simulink model "casper_counter"  (R2019a)
settings: Solver=VariableStepAuto  StartTime=0.0  StopTime=10.0  RelTol=1e-3
libraries: xbsIndex_r4 x2, xps_library x1
settings Model: Creator=talon  LastModifiedBy=talon

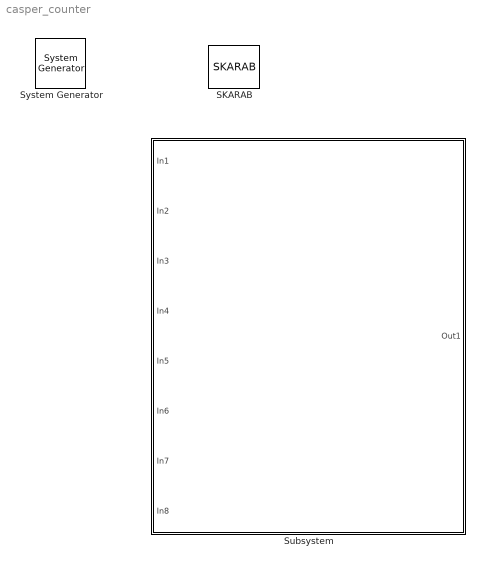
== system casper_counter ==
  " System Generator" : xbsIndex_r4/ System Generator  Tag=genX  xilinxfamily=kintex7  part=xc7k325t  speed=-3  package=fbg676  synthesis_tool=Vivado  clock_wrapper=Clock Enables  directory=./netlist  proj_type=Vivado  Synth_file=Vivado Synthesis Defaults  Impl_file=Vivado Implementation Defaults  testbench=off  simulink_period=1  sysclk_period=10  dcm_input_clock_period=10  incr_netlist=off  trim_vbits=Everywhere in SubSystem  dbl_ovrd=According to Block Masks  core_generation=According to Block Masks  run_coregen=off  deprecated_control=off  eval_field=0  block_type=sysgen
  SKARAB : xps_library/Platforms/SKARAB  Tag=xps:xsg  hw_sys=SKARAB:xc7vx690t  clk_src=sys_clk  clk_rate=156.25  sample_period=1  synthesis_tool=XST
      settings: SourceProductName=CASPER XPS Blockset
  Subsystem : Subsystem

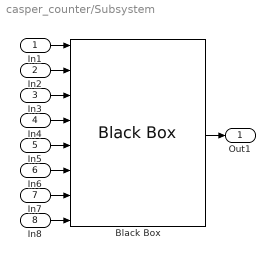
== system casper_counter/Subsystem ==
  In1 : Inport
  In2 : Inport  Port=2
  In3 : Inport  Port=3
  In4 : Inport  Port=4
  In5 : Inport  Port=5
  In6 : Inport  Port=6
  In7 : Inport  Port=7
  In8 : Inport  Port=8
  Black Box : xbsIndex_r4/Black Box  init_code=common_counter_config  sim_method=ISE Simulator  verbose=off  block_type=blackbox2
  Out1 : Outport
  wires:
  In4/1 -> Black Box/4
  In7/1 -> Black Box/7
  Black Box/1 -> Out1/1
  In3/1 -> Black Box/3
  In2/1 -> Black Box/2
  In6/1 -> Black Box/6
  In5/1 -> Black Box/5
  In8/1 -> Black Box/8
  In1/1 -> Black Box/1
